simulink model "req11"  (R2019a)
settings: Solver=FixedStepAuto  StartTime=0.0  StopTime=100  RelTol=1e-3
libraries: simulink x4
settings Model: Creator=e40014285  LastModifiedBy=e40014285
settings ConfigComp: CovEnable=on  RecordCoverage=on  CovHTMLOptions=-sRT=1 -sVT=0 -aTS=1 -bRG=1 -bTC=1 -hTR=0 -nFC=0 -nFD=1 -scm=1 -bcm=1 -xEv=0 -xEM=0  CovHtmlReporting=on  CovCumulativeReport=on  CovModelRefEnable=on  DVModelCoverageObjectives=MCDC  DVTestSuiteOptimization=Auto  DVDetectOutOfBounds=on  DVReportPDFFormat=on  DVRebuildModelRepresentation=Always

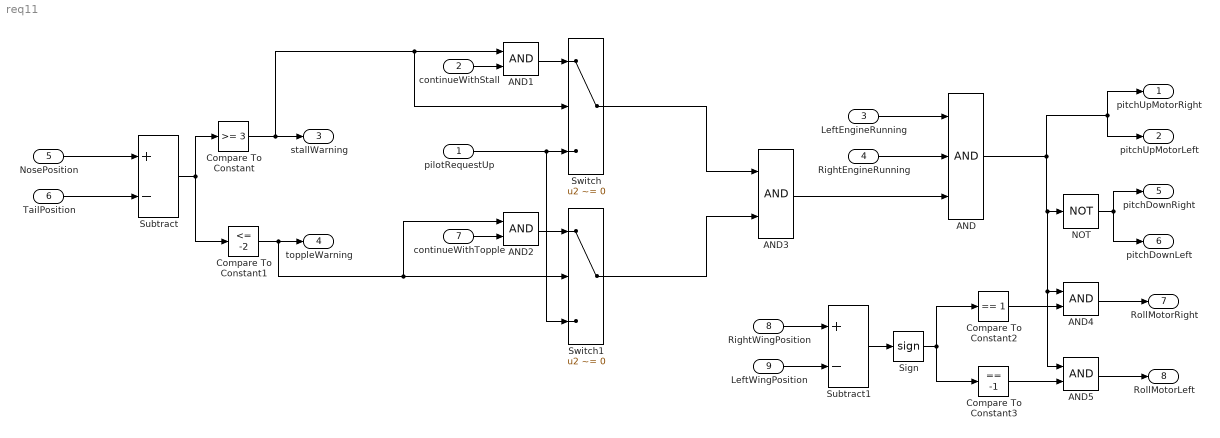
== system req11 ==
  pilotRequestUp : Inport
  continueWithStall : Inport  Port=2
  LeftEngineRunning : Inport  Port=3
  RightEngineRunning : Inport  Port=4
  NosePosition : Inport  Port=5
  TailPosition : Inport  Port=6
  continueWithTopple : Inport  Port=7
  RightWingPosition : Inport  Port=8
  LeftWingPosition : Inport  Port=9
  AND : Logic  Inputs=3  AllPortsSameDT=off  OutDataTypeStr=boolean
  AND{1..5} (5 alike) : Logic  AllPortsSameDT=off  OutDataTypeStr=boolean
  Compare To Constant : simulink/Logic and Bit Operations/Compare To Constant  relop=>=  const=3  OutDataTypeStr=boolean
  Compare To Constant1 : simulink/Logic and Bit Operations/Compare To Constant  relop=<=  const=-2  OutDataTypeStr=boolean
  Compare To Constant2 : simulink/Logic and Bit Operations/Compare To Constant  relop===  const=1  OutDataTypeStr=boolean
  Compare To Constant3 : simulink/Logic and Bit Operations/Compare To Constant  relop===  const=-1  OutDataTypeStr=boolean
  NOT : Logic  Operator=NOT  AllPortsSameDT=off  OutDataTypeStr=boolean
  Sign : Signum
  Subtract : Sum  Inputs=+-
  Subtract1 : Sum  Inputs=+-
  Switch : Switch  Criteria=u2 ~= 0
  Switch1 : Switch  Criteria=u2 ~= 0
  pitchUpMotorRight : Outport
  pitchUpMotorLeft : Outport  Port=2
  stallWarning : Outport  Port=3
  toppleWarning : Outport  Port=4
  pitchDownRight : Outport  Port=5
  pitchDownLeft : Outport  Port=6
  RollMotorRight : Outport  Port=7
  RollMotorLeft : Outport  Port=8
  wires:
  RightEngineRunning/1 -> AND/2
  LeftEngineRunning/1 -> AND/1
  NosePosition/1 -> Subtract/1
  TailPosition/1 -> Subtract/2
  Subtract/1 -> Compare To Constant1/1, Compare To Constant/1
  Compare To Constant/1 -> AND1/1, Switch/2, stallWarning/1
  continueWithStall/1 -> AND1/2
  AND1/1 -> Switch/1
  pilotRequestUp/1 -> Switch1/3, Switch/3
  continueWithTopple/1 -> AND2/2
  AND2/1 -> Switch1/1
  Compare To Constant1/1 -> AND2/1, Switch1/2, toppleWarning/1
  Switch/1 -> AND3/1
  Switch1/1 -> AND3/2
  AND3/1 -> AND/3
  AND/1 -> AND5/1, AND4/1, NOT/1, pitchUpMotorLeft/1, pitchUpMotorRight/1
  NOT/1 -> pitchDownLeft/1, pitchDownRight/1
  RightWingPosition/1 -> Subtract1/1
  LeftWingPosition/1 -> Subtract1/2
  Subtract1/1 -> Sign/1
  Sign/1 -> Compare To Constant3/1, Compare To Constant2/1
  Compare To Constant2/1 -> AND4/2
  Compare To Constant3/1 -> AND5/2
  AND4/1 -> RollMotorRight/1
  AND5/1 -> RollMotorLeft/1
